simulink model "test_blow_framebased"  (R2013a)
settings: Solver=ode45  StartTime=0.0  StopTime=100.0  RelTol=1e-3
undefined symbols (not defined in the file): dfilt, eval_time_samples, magnitude, n_pow_thres, n_sat_thres, pow_thresh_high, pow_thresh_low, sat_thresh
libraries: dsparch4 x2, etargetslib x1, instrumentlib x1
settings Model: SimulationMode=accelerator  Creator=Leonardo  LastModifiedBy=leonardo

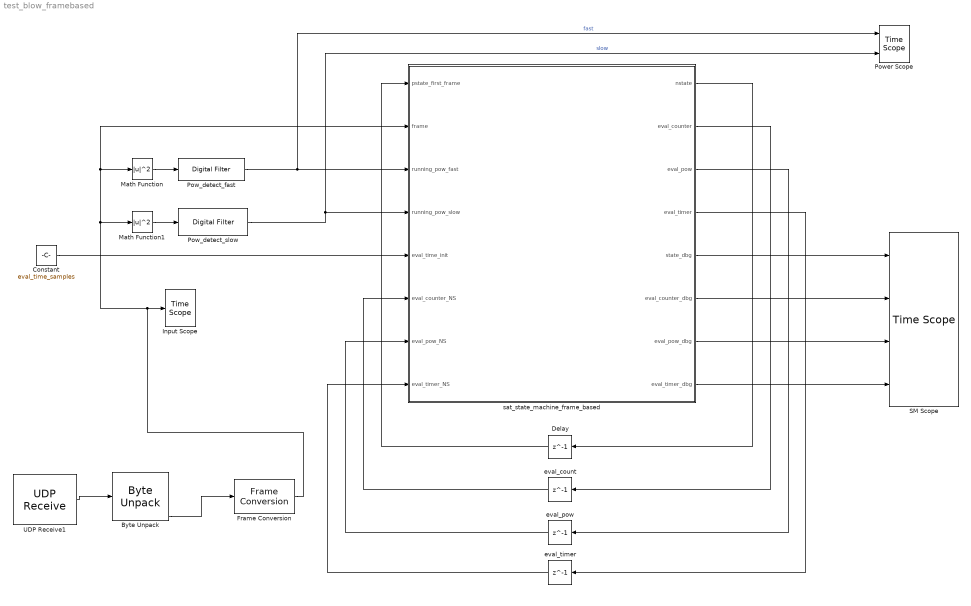
== system test_blow_framebased ==
  Byte Unpack : etargetslib/Byte Unpack  dimensions={[1],[1],[1 2],[1 2],[1],[1],[(8224-32)/4 1]}  datatypes={'int32','int32','uint32','uint32','int32','int32','single'}  byteAlign=1
  Constant : Constant  Value=eval_time_samples  OutDataTypeStr=uint32  SampleTime=Inf
  Delay : Delay  DelayLength=1  InitialCondition=uint8(1)
  Frame Conversion : FrameConversion
  Input Scope : TimeScope  DefaultConfigurationName=spbscopes.TimeScopeBlockCfg
      settings: CopyFcn=scopeextensions.ScopeBlock.callback(gcbh, 'onBlockCopy', gcbh);  DeleteFcn=scopeextensions.ScopeBlock.callback(gcbh, 'onBlockDelete');  PreSaveFcn=scopeextensions.ScopeBlock.callback(gcbh, 'onModelSave');  NameChangeFcn=scopeextensions.ScopeBlock.callback(gcbh, 'onBlockRename');  CloseFcn=scopeextensions.ScopeBlock.callback(gcbh, 'onBlockClose');  PreDeleteFcn=scopeextensions.ScopeBlock.callback(gcbh, 'onBlockPreDelete');
  Math Function : Math  Operator=magnitude^2  SaturateOnIntegerOverflow=on
  Math Function1 : Math  Operator=magnitude^2  SaturateOnIntegerOverflow=on
  Pow_detect_fast : dsparch4/Digital Filter  TypePopup=FIR (all zeros)  IIRFiltStruct=Direct form II transposed  AllPoleFiltStruct=Direct form  FIRFiltStruct=Direct form  CoeffSource=Specify via dialog  NumCoeffs=bb_fast  DenCoeffs=[1 0.1]  BiQuadCoeffs=[1 0.3 0.4 1 0.1 0.2]  LatticeCoeffs=[0.2 0.4]  denIgnore=on  FiltPerSampPopup=One filter per frame  IC=0  ICnum=0  ICden=0  roundingMode=Floor  overflowMode=off  ScaleValues=1  scaleValueFracLength=14  stageInFracLength=15  stageOutFracLength=15  FilterSource=Specify via dialog  dfiltObjectName=dfilt.dffir([1 2 1])  InputProcessing=Columns as channels (frame based)
  Pow_detect_slow : dsparch4/Digital Filter  TypePopup=FIR (all zeros)  IIRFiltStruct=Direct form II transposed  AllPoleFiltStruct=Direct form  FIRFiltStruct=Direct form  CoeffSource=Specify via dialog  NumCoeffs=bb_slow  DenCoeffs=[1 0.1]  BiQuadCoeffs=[1 0.3 0.4 1 0.1 0.2]  LatticeCoeffs=[0.2 0.4]  denIgnore=on  FiltPerSampPopup=One filter per frame  IC=0  ICnum=0  ICden=0  roundingMode=Floor  overflowMode=off  ScaleValues=1  scaleValueFracLength=14  stageInFracLength=15  stageOutFracLength=15  FilterSource=Specify via dialog  dfiltObjectName=dfilt.dffir([1 2 1])  InputProcessing=Columns as channels (frame based)
  Power Scope : TimeScope  NumInputPorts=2  DefaultConfigurationName=spbscopes.TimeScopeBlockCfg
      settings: CopyFcn=scopeextensions.ScopeBlock.callback(gcbh, 'onBlockCopy', gcbh);  DeleteFcn=scopeextensions.ScopeBlock.callback(gcbh, 'onBlockDelete');  PreSaveFcn=scopeextensions.ScopeBlock.callback(gcbh, 'onModelSave');  NameChangeFcn=scopeextensions.ScopeBlock.callback(gcbh, 'onBlockRename');  CloseFcn=scopeextensions.ScopeBlock.callback(gcbh, 'onBlockClose');  PreDeleteFcn=scopeextensions.ScopeBlock.callback(gcbh, 'onBlockPreDelete');
  SM Scope : TimeScope  NumInputPorts=4  DefaultConfigurationName=spbscopes.TimeScopeBlockCfg
      settings: CopyFcn=scopeextensions.ScopeBlock.callback(gcbh, 'onBlockCopy', gcbh);  DeleteFcn=scopeextensions.ScopeBlock.callback(gcbh, 'onBlockDelete');  PreSaveFcn=scopeextensions.ScopeBlock.callback(gcbh, 'onModelSave');  NameChangeFcn=scopeextensions.ScopeBlock.callback(gcbh, 'onBlockRename');  CloseFcn=scopeextensions.ScopeBlock.callback(gcbh, 'onBlockClose');  PreDeleteFcn=scopeextensions.ScopeBlock.callback(gcbh, 'onBlockPreDelete');
  UDP Receive1 : instrumentlib/UDP Receive  Host=192.168.1.22  Port=49782  LocalPort=50000  DataSize="[1  8224]"  EnableBlockingMode=on  Timeout=10  SampleTime=2048/44100  DataType=uint8  ByteOrder=BigEndian
  eval_count : Delay  DelayLength=1  InitialCondition=0
  eval_pow : Delay  DelayLength=1  InitialCondition=0
  eval_timer : Delay  DelayLength=1  InitialCondition=0
  sat_state_machine_frame_based : MATLAB Function  TreatAsAtomicUnit=on
  wires:
  sat_state_machine_frame_based/1(nstate) -> Delay/1
  Delay/1 -> sat_state_machine_frame_based/1(pstate_first_frame)
  Constant/1 -> sat_state_machine_frame_based/5(eval_time_init)
  Math Function/1 -> Pow_detect_fast/1
  Math Function1/1 -> Pow_detect_slow/1
  Pow_detect_fast/1 -> sat_state_machine_frame_based/3(running_pow_fast), Power Scope/1  "fast"
  Pow_detect_slow/1 -> sat_state_machine_frame_based/4(running_pow_slow), Power Scope/2  "slow"
  Frame Conversion/1 -> sat_state_machine_frame_based/2(frame), Math Function/1, Math Function1/1, Input Scope/1
  sat_state_machine_frame_based/2(eval_counter) -> eval_count/1
  eval_count/1 -> sat_state_machine_frame_based/6(eval_counter_NS)
  sat_state_machine_frame_based/4(eval_timer) -> eval_timer/1
  sat_state_machine_frame_based/3(eval_pow) -> eval_pow/1
  eval_pow/1 -> sat_state_machine_frame_based/7(eval_pow_NS)
  eval_timer/1 -> sat_state_machine_frame_based/8(eval_timer_NS)
  UDP Receive1/1 -> Byte Unpack/1
  Byte Unpack/7 -> Frame Conversion/1
  sat_state_machine_frame_based/5(state_dbg) -> SM Scope/1
  sat_state_machine_frame_based/6(eval_counter_dbg) -> SM Scope/2
  sat_state_machine_frame_based/7(eval_pow_dbg) -> SM Scope/3
  sat_state_machine_frame_based/8(eval_timer_dbg) -> SM Scope/4

== matlab function test_blow_framebased/sat_state_machine_frame_based ==
  data: pstate_first_frame input uint8; nstate output; frame input; running_pow_fast input; running_pow_slow input; pow_thresh_high parameter; pow_thresh_low parameter; sat_thresh parameter; n_sat_thres parameter; n_pow_thres parameter; eval_time_init input; eval_counter_NS input; eval_pow_NS input; eval_timer_NS input; eval_counter output uint32; eval_pow output uint32; eval_timer output uint32; state_dbg output; eval_counter_dbg output; eval_pow_dbg output; eval_timer_dbg output
function  [nstate,eval_counter,eval_pow,eval_timer,state_dbg,eval_counter_dbg,eval_pow_dbg,eval_timer_dbg] =saturation_detector(pstate_first_frame,frame,running_pow_fast,...
    running_pow_slow,pow_thresh_high,pow_thresh_low,sat_thresh,n_sat_thres,n_pow_thres,eval_time_init,...
    eval_counter_NS,eval_pow_NS,eval_timer_NS)
%#codegen

% persistent eval_counter_old;
% persistent eval_pow_old;
% persistent eval_timer_old;
% persistent frame_n_latch;
% persistent win_counter;

% State_waiting.Name='waiting'; %1
State_waiting=uint8(1);
% State_waiting.Id  = 1;
% State_evaluation.Name='evaluation';%2
% State_evaluation.Id  = 2;
State_evaluation=uint8(2);
% State_trackin.Name='trackin';%3
% State_trackin.Id  = 3;
State_trackin=uint8(3);


% if isempty(eval_counter_old)
%     eval_counter_old=0;
% end
% 
% if isempty(eval_timer_old)
%     eval_timer_old=0;
% end
% 
% if isempty(eval_pow_old)
%     eval_pow_old=0;
% end

% if isempty(win_counter)
%     win_counter=0;
% end

% running_pow_len = frame_n_latch*frame_len+sample_idx;

% switch pstate.Idpow_acc
len_frame = length(frame);

state_dbg           = uint8(zeros(len_frame,1));
eval_counter_dbg    = uint32(zeros(len_frame,1));
eval_pow_dbg        = uint32(zeros(len_frame,1));
eval_timer_dbg      = uint32(zeros(len_frame,1));

eval_pow=uint32(0);
eval_counter=uint32(0);
eval_timer=uint32(0);
nstate = uint8(0);

for sample_idx=1:len_frame
    
    sample=frame(sample_idx);
    if sample_idx==1
        eval_pow_old      = eval_pow_NS;
        eval_counter_old  = eval_counter_NS;
        eval_timer_old    = eval_timer_NS;
        pstate=pstate_first_frame;
    else
         eval_pow_old      = eval_pow;
        eval_counter_old  = eval_counter;
        eval_timer_old    = eval_timer;
        pstate = nstate;
    end

    if pstate==State_trackin
        

        if running_pow_slow(sample_idx)<=pow_thresh_low
            eval_pow=eval_pow_old+1;
        else
            eval_pow=eval_pow_old;
        end

       if eval_pow>n_pow_thres
            nstate=State_waiting;
        else
             nstate=pstate;
       end
        
       eval_counter=eval_counter_old;
       eval_timer=eval_timer_old;
        
         
%         if sample_idx==frame_len
%             frame_n_latch=frame_n_latch+1;
%         end
    
    elseif pstate==State_evaluation
        eval_timer=eval_timer_old-1;

       
        if abs(sample)>sat_thresh
            eval_counter=eval_counter_old+1;
         else
             eval_counter=eval_counter_old;
        end
        if running_pow_fast(sample_idx)>=pow_thresh_high
            eval_pow=eval_pow_old+1;
        else
            eval_pow=eval_pow_old;
        end
%         running_pow_fast=pow_acc/win_counter;

        if eval_counter>n_sat_thres && eval_timer>=0 && eval_pow>=n_pow_thres
            
            nstate=State_trackin;
            eval_pow=uint32(0);
%              running_pow_fast=(running_pow_fast*(win_counter-1)+frame)/win_counter;
%             running_pow_fast=running_pow_fast/sample_idx;

        elseif eval_timer==0

            nstate=State_waiting;
            
        else
            nstate=State_evaluation;
        end
        
%         if sample_idx==frame_len
%             frame_n_latch=frame_n_latch+1;
%         end
    
    
    elseif pstate==State_waiting
%         frame_n_latch=0;
        
        if sample>sat_thresh

            eval_timer=eval_time_init;
            eval_counter=uint32(0);
            eval_pow= uint32(0);
%              win_counter=0;
%             pow_acc=0;
            nstate=State_evaluation;
        else
            eval_timer=eval_timer_old;
             eval_counter= eval_counter_old;
             eval_pow=eval_pow_old;
            nstate=State_waiting;

        end
        
    else
        
%         pstate
        error('State Unknown');
% end
    
    
    end
    
%     eval_counter=eval_counter_old;
% eval_pow=eval_pow_old;
% eval_timer=eval_timer_old;
    
end

state_dbg(sample_idx)           =pstate;
eval_counter_dbg(sample_idx)    =eval_counter;
eval_pow_dbg(sample_idx)        =eval_pow;
eval_timer_dbg(sample_idx)      = eval_timer;
end
